simulink model "example_02"  (Simulink 8.2)
settings: Solver=FixedStepDiscrete  StartTime=0.0  StopTime=10.0  FixedStep=0.01  RelTol=1e-3
undefined symbols (not defined in the file or in its folder): sldvsubsys
libraries: sldvlib x4, simulink x3
settings Model: Creator=P  LastModifiedBy=P
settings DataIOCC: SignalLoggingSaveFormat=Dataset
settings OptimizationCC: ExpressionDepthLimit=128
settings DebuggingCC: FcnCallInpInsideContextMsg=EnableAllAsError  StateNameClashWarn=none
settings GRTTargetCC: CombineOutputUpdateFcns=on  GRTInterface=off
settings ConfigComp: Description=Design Verifier Custom Configuration Component  DVMaxProcessTime=3000  DVMaxTestCaseSteps=500  DVTestSuiteOptimization=CombinedObjectives (Nonlinear Extended)

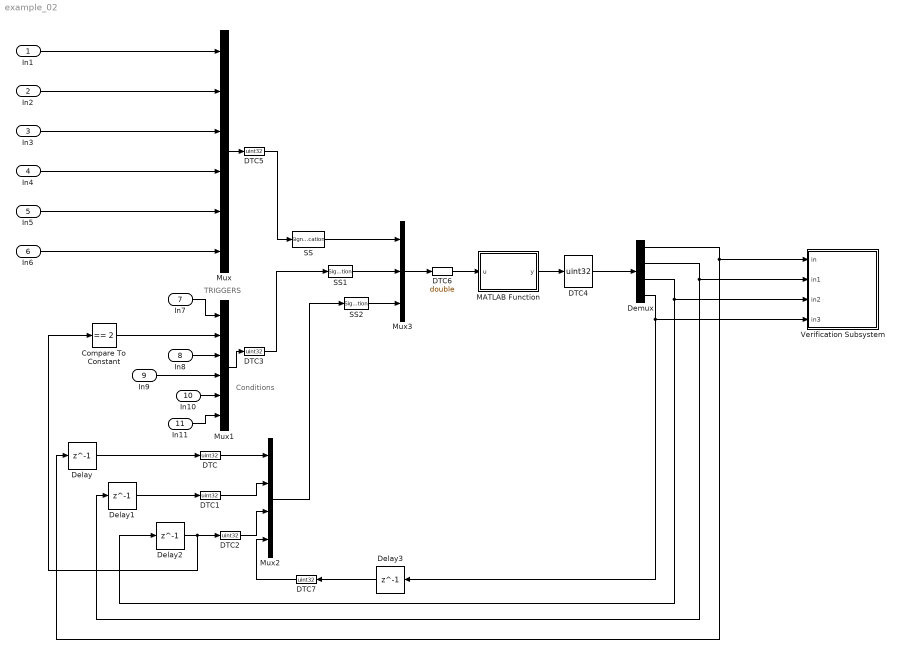
== system example_02 ==
  note: Conditions
  note: TRIGGERS
  In1 : Inport  OutDataTypeStr=boolean
  In2 : Inport  Port=2  OutDataTypeStr=boolean
  In3 : Inport  Port=3  OutDataTypeStr=boolean
  In4 : Inport  Port=4  OutDataTypeStr=boolean
  In5 : Inport  Port=5  OutDataTypeStr=boolean
  In6 : Inport  Port=6  OutDataTypeStr=boolean
  In7 : Inport  Port=7  OutDataTypeStr=boolean
  In8 : Inport  Port=8  OutDataTypeStr=boolean
  In9 : Inport  Port=9  OutDataTypeStr=boolean
  In10 : Inport  Port=10  OutDataTypeStr=boolean
  In11 : Inport  Port=11  OutDataTypeStr=boolean
  Compare To Constant : simulink/Logic and Bit Operations/Compare To Constant  relop===  const=2  OutDataTypeStr=boolean
  DTC{,1..5,7} (7 alike) : DataTypeConversion  OutDataTypeStr=uint32
  DTC6 : DataTypeConversion  OutDataTypeStr=double
  Delay{,1..3} (4 alike) : Delay  DelayLength=1  InitialCondition=1
  Demux : Demux
  MATLAB Function : MATLAB Function  TreatAsAtomicUnit=on
  Mux : Mux  Inputs=6
  Mux1 : Mux  Inputs=6
  Mux2 : Mux
  Mux3 : Mux  Inputs=3
  SS : SignalSpecification  Dimensions=6
  SS1 : SignalSpecification  Dimensions=6
  SS2 : SignalSpecification  Dimensions=4
  Verification Subsystem : Subsystem  Tag=VerificationSubsystem  DisableCoverage=on  LoadFcn=sldvsubsys('check')  TreatAsAtomicUnit=on  SimViewingDevice=on  mask(VerificationSubsystem){}
      mask init:
      | sldvsubsys('maskInit');
      settings: CopyFcn=sldvsubsys('copy');  OpenFcn=open_system(gcb,'force');
      settings: PreSaveFcn=|
      | set_param(gcb,'SimViewingDevice','on');
      | sldvsubsys('check');
      mask Help: helpview(fullfile(docroot,'toolbox','sldv','sldv.map'),'verificationsubsystem')
      mask Display: image(imread('sldvicon_versubsys.png','BackGroundColor',[1 1 1]),'center');
  wires:
  Demux/2 -> Verification Subsystem/2(in1), Delay1/1
  Delay2/1 -> Compare To Constant/1, DTC2/1
  Mux1/1 -> DTC3/1
  Delay1/1 -> DTC1/1
  Mux/1 -> DTC5/1
  Delay/1 -> DTC/1
  Mux3/1 -> DTC6/1
  Mux2/1 -> SS2/1
  Demux/1 -> Verification Subsystem/1(in), Delay/1
  In10/1 -> Mux1/5
  In3/1 -> Mux/3
  In2/1 -> Mux/2
  In4/1 -> Mux/4
  In5/1 -> Mux/5
  In6/1 -> Mux/6
  In7/1 -> Mux1/1
  In8/1 -> Mux1/3
  Compare To Constant/1 -> Mux1/2
  MATLAB Function/1(y) -> DTC4/1
  Demux/3 -> Verification Subsystem/3(in2), Delay2/1
  SS/1 -> Mux3/1
  SS1/1 -> Mux3/2
  DTC4/1 -> Demux/1
  DTC/1 -> Mux2/1
  DTC1/1 -> Mux2/2
  DTC2/1 -> Mux2/3
  DTC3/1 -> SS1/1
  SS2/1 -> Mux3/3
  DTC5/1 -> SS/1
  DTC6/1 -> MATLAB Function/1(u)
  In1/1 -> Mux/1
  In9/1 -> Mux1/4
  In11/1 -> Mux1/6
  Demux/4 -> Verification Subsystem/4(in3), Delay3/1
  DTC7/1 -> Mux2/4
  Delay3/1 -> DTC7/1

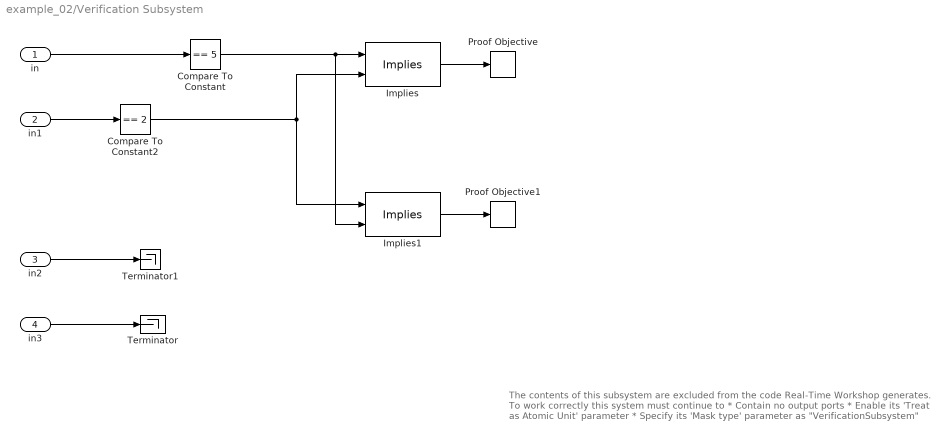
== system example_02/Verification Subsystem ==
  note: The contents of this subsystem are excluded from the code Real-Time
      | Workshop generates.
      |
      | To work correctly this system must continue to
      | * Contain no output ports
      | * Enable its 'Treat as Atomic Unit' parameter
      | * Specify its 'Mask type' parameter as "VerificationSubsystem"
  in : Inport
  in1 : Inport  Port=2
  in2 : Inport  Port=3
  in3 : Inport  Port=4
  Compare To Constant : simulink/Logic and Bit Operations/Compare To Constant  relop===  const=5  OutDataTypeStr=boolean
  Compare To Constant2 : simulink/Logic and Bit Operations/Compare To Constant  relop===  const=2  OutDataTypeStr=boolean
  Implies : sldvlib/Verification Utilities/Implies
  Implies1 : sldvlib/Verification Utilities/Implies
  Proof Objective : sldvlib/Objectives and Constraints/Proof Objective  enabled=on  customAVTBlockType=Proof Objective  intervals=true  dispValues=on  outEnabled=on  enableStopSim=off
      settings: AttributesFormatString=%<intervals>
  Proof Objective1 : sldvlib/Objectives and Constraints/Proof Objective  enabled=on  customAVTBlockType=Proof Objective  intervals=true  dispValues=on  outEnabled=on  enableStopSim=off
      settings: AttributesFormatString=%<intervals>
  Terminator : Terminator
  Terminator1 : Terminator
  wires:
  in/1 -> Compare To Constant/1
  Compare To Constant/1 -> Implies1/2, Implies/1
  Implies/1 -> Proof Objective/1
  in1/1 -> Compare To Constant2/1
  in3/1 -> Terminator/1
  in2/1 -> Terminator1/1
  Implies1/1 -> Proof Objective1/1
  Compare To Constant2/1 -> Implies1/1, Implies/2

== matlab function MATLAB Function ==
  data: u input double; y output double
function y = fcn(u)
%#codegen
nt = 6 ; nc = 6 ;
Tr = zeros(nt,1); C = zeros(nc,1);
for i = 1:nt; Tr(i) = u(i,1); end  % Assign triggers from input U
for i = 1:nc; C(i) = u(i+nt,1); end % Assign conditions from input U
M1 = u(13,1);
M2 = u(14,1);
M3 = u(15,1);
M4 = u(16,1);
% Assign the trigger to one based on priority
% Add additonal conditions to enable triggers here
TRIG = 0;
if  Tr(1) == 1, TRIG = 1;  % T1
elseif  Tr(2) == 1, TRIG = 2;  % T2
elseif  Tr(3) == 1, TRIG = 3;  % T3
elseif  Tr(4) == 1, TRIG = 4;  % T4
elseif  Tr(5) == 1, TRIG = 5;  % T5
elseif  Tr(6) == 1, TRIG = 6;  % T6
end
% 1) If in State M1_S1 AND Trigger T2 occurs THEN transit to M1_S2 if condition C3 is True
if  (M1 == 1) && (TRIG == 2) && (C(3) == 1) ; M1 = 2;
% 2) If in State M1_S2 AND Trigger T1 occurs THEN transit to M1_S1 if condition C2 is True
elseif  (M1 == 2) && (TRIG == 1) && (C(2) == 1) ; M1 = 1;
% 3) If in State M1_S2 AND Trigger T2 occurs THEN transit to M1_S4 if condition C6 is True
elseif  (M1 == 2) && (TRIG == 2) && (C(6) == 1) ; M1 = 4;
% 4) If in State M1_S2 AND Trigger T2 occurs THEN transit to M1_S3 if condition C5 is True
elseif  (M1 == 2) && (TRIG == 2) && (C(5) == 1) ; M1 = 3;
% 5) If in State M1_S2 AND Trigger T2 occurs THEN remain in M1_S2 if condition C4 is True
elseif  (M1 == 2) && (TRIG == 2) && (C(4) == 1) ; M1 = 2;
% 6) If in State M1_S2 AND Trigger T3 occurs THEN transit to M1_S4 if condition C6 is True
elseif  (M1 == 2) && (TRIG == 3) && (C(6) == 1) ; M1 = 4;
% 7) If in State M1_S2 AND Trigger T3 occurs THEN transit to M1_S3 if condition C5 is True
elseif  (M1 == 2) && (TRIG == 3) && (C(5) == 1) ; M1 = 3;
% 8) If in State M1_S2 AND Trigger T4 occurs THEN transit to M1_S3 if condition C1 is True
elseif  (M1 == 2) && (TRIG == 4) && (C(1) == 1) ; M1 = 3;
% 9) If in State M1_S2 AND Trigger T6 occurs THEN transit to M1_S3 if condition C4 is True
elseif  (M1 == 2) && (TRIG == 6) && (C(4) == 1) ; M1 = 3;
% 10) If in State M1_S3 AND Trigger T1 occurs THEN transit to M1_S1 if condition C2 is True
elseif  (M1 == 3) && (TRIG == 1) && (C(2) == 1) ; M1 = 1;
% 11) If in State M1_S3 AND Trigger T2 occurs THEN transit to M1_S2 if condition C1 is True
elseif  (M1 == 3) && (TRIG == 2) && (C(1) == 1) ; M1 = 2;
% 12) If in State M1_S3 AND Trigger T3 occurs THEN transit to M1_S2 if condition C4 is True
elseif  (M1 == 3) && (TRIG == 3) && (C(4) == 1) ; M1 = 2;
% 13) If in State M1_S3 AND Trigger T4 occurs THEN transit to M1_S4 if condition C1 is True
elseif  (M1 == 3) && (TRIG == 4) && (C(1) == 1) ; M1 = 4;
% 14) If in State M1_S4 AND Trigger T1 occurs THEN transit to M1_S1 if condition C2 is True
elseif  (M1 == 4) && (TRIG == 1) && (C(2) == 1) ; M1 = 1;
% 15) If in State M1_S4 AND Trigger T2 occurs THEN transit to M1_S2 if condition C1 is True
elseif  (M1 == 4) && (TRIG == 2) && (C(1) == 1) ; M1 = 2;
% 16) If in State M1_S4 AND Trigger T3 occurs THEN transit to M1_S2 if condition C4 is True
elseif  (M1 == 4) && (TRIG == 3) && (C(4) == 1) ; M1 = 2;
% 17) If in State M1_S4 AND Trigger T4 occurs THEN transit to M1_S5 if condition C1 is True
elseif  (M1 == 4) && (TRIG == 4) && (C(1) == 1) ; M1 = 5;
% 18) If in State M1_S5 AND Trigger T1 occurs THEN transit to M1_S1 if condition C2 is True
elseif  (M1 == 5) && (TRIG == 1) && (C(2) == 1) ; M1 = 1;
% 19) If in State M1_S5 AND Trigger T4 occurs THEN transit to M1_S2 if condition C1 is True
elseif  (M1 == 5) && (TRIG == 4) && (C(1) == 1) ; M1 = 2;
end     
%   ================================================
  
% 20) If in State M2_S1 AND Trigger T2 occurs THEN transit to M2_S2 if condition C3 is True
if  (M2 == 1) && (TRIG == 2) && (C(3) == 1) ; M2 = 2;
% 21) If in State M2_S2 AND Trigger T1 occurs THEN transit to M2_S1 if condition C2 is True
elseif  (M2 == 2) && (TRIG == 1) && (C(2) == 1) ; M2 = 1;
% 22) If in State M2_S2 AND Trigger T4 occurs THEN remain in M2_S2 if condition C1 is True
elseif  (M2 == 2) && (TRIG == 4) && (C(1) == 1) ; M2 = 2;
% 23) If in State M2_S3 AND Trigger T1 occurs THEN transit to M2_S1 if condition C2 is True
elseif  (M2 == 3) && (TRIG == 1) && (C(2) == 1) ; M2 = 1;
% 24) If in State M2_S3 AND Trigger T4 occurs THEN transit to M2_S4 if condition C1 is True
elseif  (M2 == 3) && (TRIG == 4) && (C(1) == 1) ; M2 = 4;
% 25) If in State M2_S4 AND Trigger T1 occurs THEN transit to M2_S1 if condition C2 is True
elseif  (M2 == 4) && (TRIG == 1) && (C(2) == 1) ; M2 = 1;
% 26) If in State M2_S4 AND Trigger T4 occurs THEN transit to M2_S2 if condition C1 is True
elseif  (M2 == 4) && (TRIG == 4) && (C(1) == 1) ; M2 = 2;
end     
%   ================================================
  
% 27) If in State M3_S1 AND Trigger T2 occurs THEN transit to M3_S2 if condition C3 is True
if  (M3 == 1) && (TRIG == 2) && (C(3) == 1) ; M3 = 2;
% 28) If in State M3_S1 AND Trigger T5 occurs THEN transit to M3_S2 if condition C5 is True
elseif  (M3 == 1) && (TRIG == 5) && (C(5) == 1) ; M3 = 2;
% 29) If in State M3_S2 AND Trigger T1 occurs THEN transit to M3_S1 if condition C2 is True
elseif  (M3 == 2) && (TRIG == 1) && (C(2) == 1) ; M3 = 1;
% 30) If in State M3_S2 AND Trigger T5 occurs THEN transit to M3_S1 if condition C1 is True
elseif  (M3 == 2) && (TRIG == 5) && (C(1) == 1) ; M3 = 1;
end     
%   ================================================
  
% 31) If in State M4_S1 AND Trigger T2 occurs THEN transit to M4_S2 if condition C3 is True
if  (M4 == 1) && (TRIG == 2) && (C(3) == 1) ; M4 = 2;
% 32) If in State M4_S1 AND Trigger T5 occurs THEN transit to M4_S2 if condition C6 is True
elseif  (M4 == 1) && (TRIG == 5) && (C(6) == 1) ; M4 = 2;
% 33) If in State M4_S2 AND Trigger T1 occurs THEN transit to M4_S1 if condition C2 is True
elseif  (M4 == 2) && (TRIG == 1) && (C(2) == 1) ; M4 = 1;
% 34) If in State M4_S2 AND Trigger T5 occurs THEN transit to M4_S1 if condition C1 is True
elseif  (M4 == 2) && (TRIG == 5) && (C(1) == 1) ; M4 = 1;
end     
%   ================================================
  
% ============== Set the outputs ===========
y = zeros(4,1);
y(1) = M1;
y(2) = M2;
y(3) = M3;
y(4) = M4;
